simulink model "Sample2"  (R2018b)
settings: Solver=FixedStepAuto  StartTime=0.0  StopTime=10.0  FixedStep=0.1  RelTol=1e-3
settings Model: Creator=Amir  LastModifiedBy=Amir

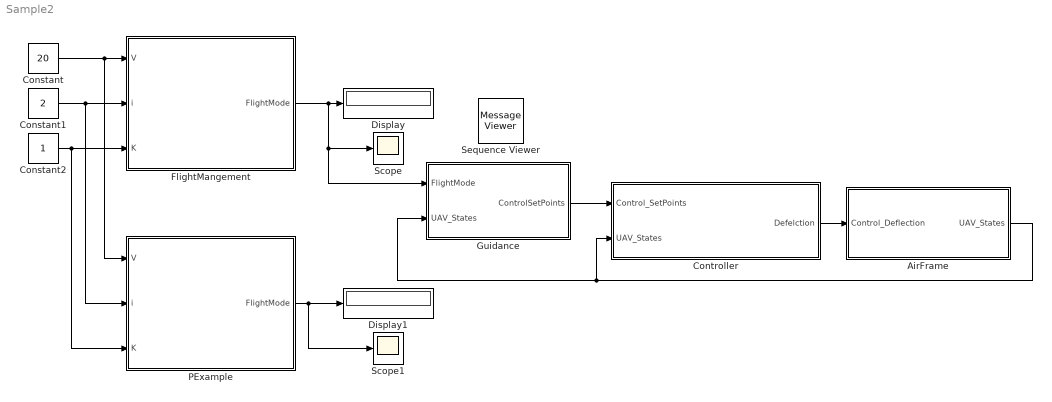
== system Sample2 ==
  AirFrame : Subsystem
  Constant : Constant  Value=20
  Constant1 : Constant  Value=2
  Constant2 : Constant
  Controller : Subsystem
  Display : Display
  Display1 : Display
  FlightMangement : Stateflow chart  TreatAsAtomicUnit=on
  Guidance : Stateflow chart  TreatAsAtomicUnit=on
  PExample : Stateflow chart  TreatAsAtomicUnit=on
  Scope : Scope
  Scope1 : Scope
  Sequence Viewer : MessageViewer
  wires:
  Constant/1 -> PExample/1(V), FlightMangement/1(V)
  Constant1/1 -> PExample/2(i), FlightMangement/2(i)
  FlightMangement/1(FlightMode) -> Guidance/1(FlightMode), Scope/1, Display/1
  Constant2/1 -> PExample/3(K), FlightMangement/3(K)
  PExample/1(FlightMode) -> Scope1/1, Display1/1
  Controller/1(Defelction) -> AirFrame/1(Control_Deflection)
  AirFrame/1(UAV_States) -> Controller/2(UAV_States), Guidance/2(UAV_States)
  Guidance/1(ControlSetPoints) -> Controller/1(Control_SetPoints)

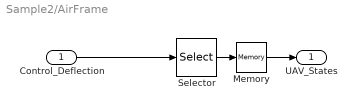
== system Sample2/AirFrame ==
  Control_Deflection : Inport
  Memory : Memory
  Selector : Selector  InputPortWidth=4  IndexOptions=Index vector (dialog)  Indices=1  OutputSizes=1
  UAV_States : Outport
  wires:
  Control_Deflection/1 -> Selector/1
  Selector/1 -> Memory/1
  Memory/1 -> UAV_States/1

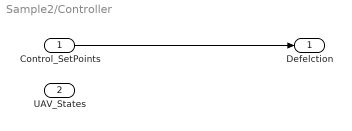
== system Sample2/Controller ==
  Control_SetPoints : Inport
  UAV_States : Inport  Port=2
  Defelction : Outport
  wires:
  Control_SetPoints/1 -> Defelction/1

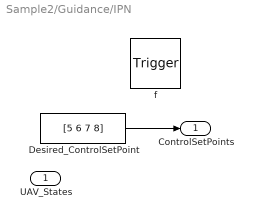
== system Sample2/Guidance/IPN ==
  UAV_States : Inport  OutDataTypeStr=double  PortDimensions=1
  f : TriggerPort  TriggerType=function-call  VariantControl=(inherit)
      settings: CopyFcn=Stateflow.SLINSF.SimulinkMan.removeBlockPreDeleteFcn  PreDeleteFcn=Stateflow.SLINSF.SimulinkMan.unsafePredeleteFcn
  Desired_ControlSetPoint : Constant  Value=[5 6 7 8]
  ControlSetPoints : Outport
  wires:
  Desired_ControlSetPoint/1 -> ControlSetPoints/1

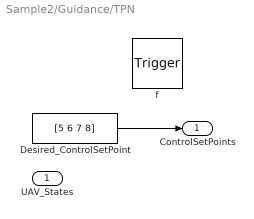
== system Sample2/Guidance/TPN ==
  UAV_States : Inport  OutDataTypeStr=double  PortDimensions=1
  f : TriggerPort  TriggerType=function-call  VariantControl=(inherit)
      settings: CopyFcn=Stateflow.SLINSF.SimulinkMan.removeBlockPreDeleteFcn  PreDeleteFcn=Stateflow.SLINSF.SimulinkMan.unsafePredeleteFcn
  Desired_ControlSetPoint : Constant  Value=[5 6 7 8]
  ControlSetPoints : Outport
  wires:
  Desired_ControlSetPoint/1 -> ControlSetPoints/1

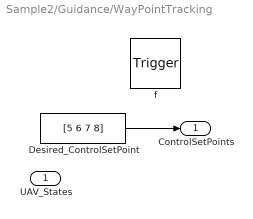
== system Sample2/Guidance/WayPointTracking ==
  UAV_States : Inport  OutDataTypeStr=double  PortDimensions=1
  f : TriggerPort  TriggerType=function-call  VariantControl=(inherit)
      settings: CopyFcn=Stateflow.SLINSF.SimulinkMan.removeBlockPreDeleteFcn  PreDeleteFcn=Stateflow.SLINSF.SimulinkMan.unsafePredeleteFcn
  Desired_ControlSetPoint : Constant  Value=[5 6 7 8]
  ControlSetPoints : Outport
  wires:
  Desired_ControlSetPoint/1 -> ControlSetPoints/1

== stateflow chart Sample2/PExample ==
  state Loiter [parallel]
    en:
    if i==2
    FlightMode=4;
    else
    FlightMode=6;
    end
    du:
    if i==2
    FlightMode=5;
    else
    FlightMode=7;
    end
    settings: executionOrder=1
  state WayPoint [parallel]
    if i==2
    FlightMode=3;
    else
    FlightMode=9;
    end
    settings: executionOrder=3
  state Cruise [parallel]
    if i==1
    FlightMode=5;
    else
    FlightMode=8;
    end
    settings: executionOrder=2
  data: FlightMode output; V input; i input; K input

== stateflow chart Sample2/Guidance ==
  state GuidanceMethodSelector
    switch FlightMode
    case 8
    ControlSetPoints = TPN(UAV_States)
    case 4
    ControlSetPoints = IPN(UAV_States)
    case 5
    ControlSetPoints = WayPointTracking(UAV_States)
    end
  state ControlSetPoints = IPN(UAV_States) [function]
  state ControlSetPoints = TPN(UAV_States) [function]
  state ControlSetPoints = WayPointTracking(UAV_States) [function]
  (default) -> GuidanceMethodSelector
  data: ControlSetPoints function_output; UAV_States function_input double size=1; ControlSetPoints function_output; UAV_States function_input double size=1; ControlSetPoints function_output; UAV_States function_input double size=1; FlightMode input; UAV_States input; ControlSetPoints output

== stateflow chart Sample2/FlightMangement ==
  state Flighter
    state Loiter
      en:
      if i==2
      FlightMode=4;
      else
      FlightMode=6;
      end
      du:
      if i==2
      FlightMode=5;
      else
      FlightMode=7;
      end
    state Cruise
      if i==1
      FlightMode=5;
      else
      FlightMode=8;
      end
    state WayPoint
      if i==2
      FlightMode=3;
      else
      FlightMode=9;
      end
    (default) -> Cruise
    Cruise -> Loiter [order 2] : [V<30]
    Loiter -> Cruise [order 1] : [V>=30]
    Cruise -> WayPoint [order 1] : [V>40]
    WayPoint -> Cruise [order 2] : [V<=40]
    Loiter -> WayPoint [order 2] : [K~=1]
    WayPoint -> Loiter [order 1] : [K==1]
  (default) -> Flighter
  data: FlightMode output; V input; i input; K input
